simulink model "adm_pcie_9h7_dts_dual_2x100g_dsp"  (R2019a)
settings: Solver=VariableStepAuto  StartTime=0.0  StopTime=10.0  RelTol=1e-3
undefined symbols (not defined in the file): datetime, posixtime
libraries: xbsIndex_r4 x7868, casper_library_misc x12, xps_library x9
(part 4 of 65)

== system adm_pcie_9h7_dts_dual_2x100g_dsp/pipeline0/eq/core5 ==
  note: make up for lack
      | of final FFT reorder
  sync : Inport
  in : Inport  Port=2
  Concat : xbsIndex_r4/Concat  num_inputs=8  dbl_ovrd=off  block_type=concat
  Constant : xbsIndex_r4/Constant  const=1  gui_display_data_type=Boolean  arith_type=Boolean  n_bits=16  bin_pt=14  preci_type=Single  exp_width=8  frac_width=24  explicit_period=on  period=1  equ=P=C  opselect=C  inp2=PCIN>>17  opr=+  inp1=P  carry=CIN  dbl_ovrd=off  block_type=constant
  Constant4 : xbsIndex_r4/Constant  const=0  gui_display_data_type=Fixed-point  arith_type=Unsigned  n_bits=18  bin_pt=0  preci_type=Single  exp_width=8  frac_width=24  explicit_period=on  period=1  equ=P=C  opselect=C  inp2=PCIN>>17  opr=+  inp1=P  carry=CIN  dbl_ovrd=off  block_type=constant
  Constant5 : xbsIndex_r4/Constant  const=0  gui_display_data_type=Fixed-point  arith_type=Boolean  n_bits=1  bin_pt=0  preci_type=Single  exp_width=8  frac_width=24  explicit_period=on  period=1  equ=P=C  opselect=C  inp2=PCIN>>17  opr=+  inp1=P  carry=CIN  dbl_ovrd=off  block_type=constant
  Counter : xbsIndex_r4/Counter  cnt_type=Count Limited  cnt_to=2^nchan * nants - 1  operation=Up  start_count=0  cnt_by_val=1  arith_type=Unsigned  n_bits=ceil(log2(2^nchan * nants))  bin_pt=0  load_pin=off  rst=on  en=off  explicit_period=off  period=1  use_behavioral_HDL=off  implementation=Fabric  use_rpm=on  dbl_ovrd=off  block_type=counter
      settings: xl_area=[0, 0, 0, 0, 0, 0, 0]
  Counter1 : xbsIndex_r4/Counter  cnt_type=Free Running  cnt_to=Inf  operation=Up  start_count=0  cnt_by_val=1  arith_type=Unsigned  n_bits=32  bin_pt=0  load_pin=off  rst=on  en=on  explicit_period=on  period=1  use_behavioral_HDL=off  implementation=Fabric  dbl_ovrd=off  block_type=counter
  Delay2 : xbsIndex_r4/Delay  rst=off  infoeditControl=Selection of Reset will increase slice count due to use of real FFs and instead of SRLs  en=off  latency=1  reg_retiming=on  dbl_ovrd=off  block_type=delay
      settings: xl_area=[0, 0, 0, 0, 0, 0, 0]
  Delay4 : xbsIndex_r4/Delay  rst=off  infoeditControl=Selection of Reset will increase slice count due to use of real FFs and instead of SRLs  en=off  latency=6  reg_retiming=on  dbl_ovrd=off  block_type=delay
      settings: xl_area=[0, 0, 0, 0, 0, 0, 0]
  Delay5 : xbsIndex_r4/Delay  rst=off  infoeditControl=Selection of Reset will increase slice count due to use of real FFs and instead of SRLs  en=off  latency=1  reg_retiming=on  dbl_ovrd=off  block_type=delay
      settings: xl_area=[0, 0, 0, 0, 0, 0, 0]
  Logical : xbsIndex_r4/Logical  logical_function=OR  inputs=8  en=off  latency=1  precision=Full  arith_type=Unsigned  n_bits=16  bin_pt=0  align_bp=on  dbl_ovrd=off  block_type=logical
  bus_expand4 : Subsystem  AncestorBlock=casper_library_flow_control/bus_expand  mask(bus_expand){mode=divisions of equal size, outputNum=8, outputWidth=18*2, outputBinaryPt=0, outputArithmeticType=0, show_format=off, outputToWorkspace=off, variablePrefix=out, outputToModelAsWell=on}
      mask prompts: outputNum "Number of outputs:"; outputWidth "Output width:"; outputBinaryPt "Output binary point position:"; outputArithmeticType "Output arithmetic type (ufix=0, fix=1, bool=2):"; show_format "Print format string?"; outputToWorkspace "Output to workspace?"; variablePrefix "Variable name prefix:"; outputToModelAsWell "Output to model as well?"
      mask help:
      | Expands a 'bus' made using a bus_create or Xilinx
      | concat block.
      | The input will be divided into the specified number
      | of outputs with the specified arithmetic types.
      | Divisions are made from most significant bit.
      mask init: same as adm_pcie_9h7_dts_dual_2x100g_dsp/pipeline0/eq/bus_expand4
      settings: AttributesFormatString=8 outputs
      mask TypeOptions mode: divisions of equal size | divisions of arbitrary size
      mask Callback mode: bus_expand_callback();
      mask Callback outputWidth: bus_expand_callback();
      mask Callback outputToWorkspace: bus_expand_callback();
  clip_cnt : Subsystem  Tag=xps:sw_reg  AncestorBlock=xps_library/Memory/software_register  mask(swreg){io_dir=To Processor, io_delay=0, init_val=0, sample_period=1, names=reg, bitwidths=32, bin_pts=0, arith_types=0, sim_port=on, show_format=on, desc_str=}
      mask prompts: io_dir "I/O direction"; io_delay "I/O delay"; init_val "Initial Value"; sample_period "Sample period"; names "Bitfield names [msb...lsb]"; bitwidths "Bitfield widths"; bin_pts "Bitfield binary pts"; arith_types "Bitfield types, ufix=0, fix=1, bool=2"; sim_port "Provide sim input/output?"; show_format "Print format string?"; desc_str "Description"
      mask help: A 32-bit software-accessible register. Can be divided into bitfields of varying widths and types using the fields in the block mask.
      mask init:
      | swreg_init(gcb)
      settings: AttributesFormatString=1output:uf32.0 = 32 bits
      mask TypeOptions io_dir: To Processor | From Processor
      mask Callback io_dir:
      | mask_enables = get_param(gcb, 'MaskEnables');
      | mask_names = get_param(gcb, 'MaskNames');
      | if strcmp(get_param(gcb, 'io_dir'), 'To Processor'),
      |     mask_enables{ismember(mask_names, 'sample_period')} = 'off';
      | else
      |     mask_enables{ismember(mask_names, 'sample_period')} = 'on';
      | end
      | set_param(gcb, 'MaskEnables', mask_enables);
      mask DialogControl ParameterTabVar0 Prompt: Setup
  coeffs : Subsystem  Tag=xps:bram  AncestorBlock=xps_library/Memory/shared_bram  mask{sample_rate=1, init_vals=[0:2^10-1], data_bin_pt=0, optimization=Minimum_Area, reg_core_output=off, reg_prim_output=off, data_width=16, addr_width=ceil(log2(2^nchan * nants)), arith_type=Unsigned, desc_str=|, type_desc=uint16}
      mask desc_str=|
      | For register name suffix ``<n>_coeffs``, this
      | memory holds coefficients for F-engine streams
      | ``16n..16(n+1)-1``. Coefficients are stored
      | as a ``[16, n_fft_channels / 8]`` array, where the first
      | axis (over input number) varies *slowest*.
      | Coefficients are shared over 8 consecutive frequency
      | channels, with coefficient ``m`` being applied to
      | frequency channel ``m..8(m+1)-1``. Coefficients
      | are interpretted with 5 bits below the binary point.
      mask prompts: sample_rate "Sample rate"; init_vals "Initial values (simulation only)"; data_bin_pt "Data Binary Point"; reg_core_output "Register Core Output"; reg_prim_output "Register Primitive Output"; data_width "Data Width"; addr_width "Address width"; arith_type "Output Data Type"; desc_str "Description"; type_desc "Word Type Description"
      mask init:
      | shared_bram_mask;
      mask TypeOptions optimization: Minimum_Area | Low_Power
      mask TypeOptions data_width: 8 | 16 | 32 | 64 | 128
      mask TypeOptions arith_type: Unsigned | Signed  (2's comp)
      mask DialogControl Container4 Prompt: Configuration
      mask DialogControl Container10 Prompt: Documentation
  round1 : Subsystem
      settings: AttributesFormatString=latency=5
  round2 : Subsystem
      settings: AttributesFormatString=latency=5
  round3 : Subsystem
      settings: AttributesFormatString=latency=5
  round4 : Subsystem
      settings: AttributesFormatString=latency=5
  round5 : Subsystem
      settings: AttributesFormatString=latency=5
  round6 : Subsystem
      settings: AttributesFormatString=latency=5
  round7 : Subsystem
      settings: AttributesFormatString=latency=5
  round8 : Subsystem
      settings: AttributesFormatString=latency=5
  sync_out : Outport
  dout : Outport  Port=2
  wires:
  Delay5/1 -> Delay4/1
  Delay2/1 -> bus_expand4/1(bus_in)
  coeffs/1(data_out) -> round8/2(scale), round7/2(scale), round6/2(scale), round5/2(scale), round4/2(scale), round3/2(scale), round2/2(scale), round1/2(scale)
  in/1 -> Delay2/1
  sync/1 -> Delay5/1, Counter/1
  Constant5/1 -> coeffs/3(we)
  Constant4/1 -> coeffs/2(data_in)
  bus_expand4/3(out6) -> round3/1(din)
  bus_expand4/2(out7) -> round2/1(din)
  bus_expand4/1(msb_out8) -> round1/1(din)
  bus_expand4/4(out5) -> round4/1(din)
  bus_expand4/5(out4) -> round5/1(din)
  bus_expand4/6(out3) -> round6/1(din)
  bus_expand4/7(out2) -> round7/1(din)
  bus_expand4/8(lsb_out1) -> round8/1(din)
  round1/1(dout) -> Concat/1
  round2/1(dout) -> Concat/2
  round3/1(dout) -> Concat/3
  round4/1(dout) -> Concat/4
  round5/1(dout) -> Concat/5
  round6/1(dout) -> Concat/6
  round7/1(dout) -> Concat/7
  round8/1(dout) -> Concat/8
  round1/2(clip) -> Logical/1
  round3/2(clip) -> Logical/3
  round2/2(clip) -> Logical/2
  round6/2(clip) -> Logical/6
  round5/2(clip) -> Logical/5
  round7/2(clip) -> Logical/7
  Logical/1 -> Counter1/2
  round4/2(clip) -> Logical/4
  Counter1/1 -> clip_cnt/1(out_reg)
  round8/2(clip) -> Logical/8
  Concat/1 -> dout/1
  Delay4/1 -> sync_out/1, Counter1/1
  Constant/1 -> ?
  Counter/1 -> coeffs/1(addr)

== system adm_pcie_9h7_dts_dual_2x100g_dsp/pipeline0/eq/core6 ==
  note: make up for lack
      | of final FFT reorder
  sync : Inport
  in : Inport  Port=2
  Concat : xbsIndex_r4/Concat  num_inputs=8  dbl_ovrd=off  block_type=concat
  Constant : xbsIndex_r4/Constant  const=1  gui_display_data_type=Boolean  arith_type=Boolean  n_bits=16  bin_pt=14  preci_type=Single  exp_width=8  frac_width=24  explicit_period=on  period=1  equ=P=C  opselect=C  inp2=PCIN>>17  opr=+  inp1=P  carry=CIN  dbl_ovrd=off  block_type=constant
  Constant4 : xbsIndex_r4/Constant  const=0  gui_display_data_type=Fixed-point  arith_type=Unsigned  n_bits=18  bin_pt=0  preci_type=Single  exp_width=8  frac_width=24  explicit_period=on  period=1  equ=P=C  opselect=C  inp2=PCIN>>17  opr=+  inp1=P  carry=CIN  dbl_ovrd=off  block_type=constant
  Constant5 : xbsIndex_r4/Constant  const=0  gui_display_data_type=Fixed-point  arith_type=Boolean  n_bits=1  bin_pt=0  preci_type=Single  exp_width=8  frac_width=24  explicit_period=on  period=1  equ=P=C  opselect=C  inp2=PCIN>>17  opr=+  inp1=P  carry=CIN  dbl_ovrd=off  block_type=constant
  Counter : xbsIndex_r4/Counter  cnt_type=Count Limited  cnt_to=2^nchan * nants - 1  operation=Up  start_count=0  cnt_by_val=1  arith_type=Unsigned  n_bits=ceil(log2(2^nchan * nants))  bin_pt=0  load_pin=off  rst=on  en=off  explicit_period=off  period=1  use_behavioral_HDL=off  implementation=Fabric  use_rpm=on  dbl_ovrd=off  block_type=counter
      settings: xl_area=[0, 0, 0, 0, 0, 0, 0]
  Counter1 : xbsIndex_r4/Counter  cnt_type=Free Running  cnt_to=Inf  operation=Up  start_count=0  cnt_by_val=1  arith_type=Unsigned  n_bits=32  bin_pt=0  load_pin=off  rst=on  en=on  explicit_period=on  period=1  use_behavioral_HDL=off  implementation=Fabric  dbl_ovrd=off  block_type=counter
  Delay2 : xbsIndex_r4/Delay  rst=off  infoeditControl=Selection of Reset will increase slice count due to use of real FFs and instead of SRLs  en=off  latency=1  reg_retiming=on  dbl_ovrd=off  block_type=delay
      settings: xl_area=[0, 0, 0, 0, 0, 0, 0]
  Delay4 : xbsIndex_r4/Delay  rst=off  infoeditControl=Selection of Reset will increase slice count due to use of real FFs and instead of SRLs  en=off  latency=6  reg_retiming=on  dbl_ovrd=off  block_type=delay
      settings: xl_area=[0, 0, 0, 0, 0, 0, 0]
  Delay5 : xbsIndex_r4/Delay  rst=off  infoeditControl=Selection of Reset will increase slice count due to use of real FFs and instead of SRLs  en=off  latency=1  reg_retiming=on  dbl_ovrd=off  block_type=delay
      settings: xl_area=[0, 0, 0, 0, 0, 0, 0]
  Logical : xbsIndex_r4/Logical  logical_function=OR  inputs=8  en=off  latency=1  precision=Full  arith_type=Unsigned  n_bits=16  bin_pt=0  align_bp=on  dbl_ovrd=off  block_type=logical
  bus_expand4 : Subsystem  AncestorBlock=casper_library_flow_control/bus_expand  mask(bus_expand){mode=divisions of equal size, outputNum=8, outputWidth=18*2, outputBinaryPt=0, outputArithmeticType=0, show_format=off, outputToWorkspace=off, variablePrefix=out, outputToModelAsWell=on}
      mask prompts: outputNum "Number of outputs:"; outputWidth "Output width:"; outputBinaryPt "Output binary point position:"; outputArithmeticType "Output arithmetic type (ufix=0, fix=1, bool=2):"; show_format "Print format string?"; outputToWorkspace "Output to workspace?"; variablePrefix "Variable name prefix:"; outputToModelAsWell "Output to model as well?"
      mask help:
      | Expands a 'bus' made using a bus_create or Xilinx
      | concat block.
      | The input will be divided into the specified number
      | of outputs with the specified arithmetic types.
      | Divisions are made from most significant bit.
      mask init: same as adm_pcie_9h7_dts_dual_2x100g_dsp/pipeline0/eq/bus_expand4
      settings: AttributesFormatString=8 outputs
      mask TypeOptions mode: divisions of equal size | divisions of arbitrary size
      mask Callback mode: bus_expand_callback();
      mask Callback outputWidth: bus_expand_callback();
      mask Callback outputToWorkspace: bus_expand_callback();
  clip_cnt : Subsystem  Tag=xps:sw_reg  AncestorBlock=xps_library/Memory/software_register  mask(swreg){io_dir=To Processor, io_delay=0, init_val=0, sample_period=1, names=reg, bitwidths=32, bin_pts=0, arith_types=0, sim_port=on, show_format=on, desc_str=}
      mask prompts: io_dir "I/O direction"; io_delay "I/O delay"; init_val "Initial Value"; sample_period "Sample period"; names "Bitfield names [msb...lsb]"; bitwidths "Bitfield widths"; bin_pts "Bitfield binary pts"; arith_types "Bitfield types, ufix=0, fix=1, bool=2"; sim_port "Provide sim input/output?"; show_format "Print format string?"; desc_str "Description"
      mask help: A 32-bit software-accessible register. Can be divided into bitfields of varying widths and types using the fields in the block mask.
      mask init:
      | swreg_init(gcb)
      settings: AttributesFormatString=1output:uf32.0 = 32 bits
      mask TypeOptions io_dir: To Processor | From Processor
      mask Callback io_dir:
      | mask_enables = get_param(gcb, 'MaskEnables');
      | mask_names = get_param(gcb, 'MaskNames');
      | if strcmp(get_param(gcb, 'io_dir'), 'To Processor'),
      |     mask_enables{ismember(mask_names, 'sample_period')} = 'off';
      | else
      |     mask_enables{ismember(mask_names, 'sample_period')} = 'on';
      | end
      | set_param(gcb, 'MaskEnables', mask_enables);
      mask DialogControl ParameterTabVar0 Prompt: Setup
  coeffs : Subsystem  Tag=xps:bram  AncestorBlock=xps_library/Memory/shared_bram  mask{sample_rate=1, init_vals=[0:2^10-1], data_bin_pt=0, optimization=Minimum_Area, reg_core_output=off, reg_prim_output=off, data_width=16, addr_width=ceil(log2(2^nchan * nants)), arith_type=Unsigned, desc_str=|, type_desc=uint16}
      mask desc_str=|
      | For register name suffix ``<n>_coeffs``, this
      | memory holds coefficients for F-engine streams
      | ``16n..16(n+1)-1``. Coefficients are stored
      | as a ``[16, n_fft_channels / 8]`` array, where the first
      | axis (over input number) varies *slowest*.
      | Coefficients are shared over 8 consecutive frequency
      | channels, with coefficient ``m`` being applied to
      | frequency channel ``m..8(m+1)-1``. Coefficients
      | are interpretted with 5 bits below the binary point.
      mask prompts: sample_rate "Sample rate"; init_vals "Initial values (simulation only)"; data_bin_pt "Data Binary Point"; reg_core_output "Register Core Output"; reg_prim_output "Register Primitive Output"; data_width "Data Width"; addr_width "Address width"; arith_type "Output Data Type"; desc_str "Description"; type_desc "Word Type Description"
      mask init:
      | shared_bram_mask;
      mask TypeOptions optimization: Minimum_Area | Low_Power
      mask TypeOptions data_width: 8 | 16 | 32 | 64 | 128
      mask TypeOptions arith_type: Unsigned | Signed  (2's comp)
      mask DialogControl Container4 Prompt: Configuration
      mask DialogControl Container10 Prompt: Documentation
  round1 : Subsystem
      settings: AttributesFormatString=latency=5
  round2 : Subsystem
      settings: AttributesFormatString=latency=5
  round3 : Subsystem
      settings: AttributesFormatString=latency=5
  round4 : Subsystem
      settings: AttributesFormatString=latency=5
  round5 : Subsystem
      settings: AttributesFormatString=latency=5
  round6 : Subsystem
      settings: AttributesFormatString=latency=5
  round7 : Subsystem
      settings: AttributesFormatString=latency=5
  round8 : Subsystem
      settings: AttributesFormatString=latency=5
  sync_out : Outport
  dout : Outport  Port=2
  wires:
  Delay5/1 -> Delay4/1
  Delay2/1 -> bus_expand4/1(bus_in)
  coeffs/1(data_out) -> round8/2(scale), round7/2(scale), round6/2(scale), round5/2(scale), round4/2(scale), round3/2(scale), round2/2(scale), round1/2(scale)
  in/1 -> Delay2/1
  sync/1 -> Delay5/1, Counter/1
  Constant5/1 -> coeffs/3(we)
  Constant4/1 -> coeffs/2(data_in)
  bus_expand4/3(out6) -> round3/1(din)
  bus_expand4/2(out7) -> round2/1(din)
  bus_expand4/1(msb_out8) -> round1/1(din)
  bus_expand4/4(out5) -> round4/1(din)
  bus_expand4/5(out4) -> round5/1(din)
  bus_expand4/6(out3) -> round6/1(din)
  bus_expand4/7(out2) -> round7/1(din)
  bus_expand4/8(lsb_out1) -> round8/1(din)
  round1/1(dout) -> Concat/1
  round2/1(dout) -> Concat/2
  round3/1(dout) -> Concat/3
  round4/1(dout) -> Concat/4
  round5/1(dout) -> Concat/5
  round6/1(dout) -> Concat/6
  round7/1(dout) -> Concat/7
  round8/1(dout) -> Concat/8
  round1/2(clip) -> Logical/1
  round3/2(clip) -> Logical/3
  round2/2(clip) -> Logical/2
  round6/2(clip) -> Logical/6
  round5/2(clip) -> Logical/5
  round7/2(clip) -> Logical/7
  Logical/1 -> Counter1/2
  round4/2(clip) -> Logical/4
  Counter1/1 -> clip_cnt/1(out_reg)
  round8/2(clip) -> Logical/8
  Concat/1 -> dout/1
  Delay4/1 -> sync_out/1, Counter1/1
  Constant/1 -> ?
  Counter/1 -> coeffs/1(addr)

== system adm_pcie_9h7_dts_dual_2x100g_dsp/pipeline0/eq/core7 ==
  note: make up for lack
      | of final FFT reorder
  sync : Inport
  in : Inport  Port=2
  Concat : xbsIndex_r4/Concat  num_inputs=8  dbl_ovrd=off  block_type=concat
  Constant : xbsIndex_r4/Constant  const=1  gui_display_data_type=Boolean  arith_type=Boolean  n_bits=16  bin_pt=14  preci_type=Single  exp_width=8  frac_width=24  explicit_period=on  period=1  equ=P=C  opselect=C  inp2=PCIN>>17  opr=+  inp1=P  carry=CIN  dbl_ovrd=off  block_type=constant
  Constant4 : xbsIndex_r4/Constant  const=0  gui_display_data_type=Fixed-point  arith_type=Unsigned  n_bits=18  bin_pt=0  preci_type=Single  exp_width=8  frac_width=24  explicit_period=on  period=1  equ=P=C  opselect=C  inp2=PCIN>>17  opr=+  inp1=P  carry=CIN  dbl_ovrd=off  block_type=constant
  Constant5 : xbsIndex_r4/Constant  const=0  gui_display_data_type=Fixed-point  arith_type=Boolean  n_bits=1  bin_pt=0  preci_type=Single  exp_width=8  frac_width=24  explicit_period=on  period=1  equ=P=C  opselect=C  inp2=PCIN>>17  opr=+  inp1=P  carry=CIN  dbl_ovrd=off  block_type=constant
  Counter : xbsIndex_r4/Counter  cnt_type=Count Limited  cnt_to=2^nchan * nants - 1  operation=Up  start_count=0  cnt_by_val=1  arith_type=Unsigned  n_bits=ceil(log2(2^nchan * nants))  bin_pt=0  load_pin=off  rst=on  en=off  explicit_period=off  period=1  use_behavioral_HDL=off  implementation=Fabric  use_rpm=on  dbl_ovrd=off  block_type=counter
      settings: xl_area=[0, 0, 0, 0, 0, 0, 0]
  Counter1 : xbsIndex_r4/Counter  cnt_type=Free Running  cnt_to=Inf  operation=Up  start_count=0  cnt_by_val=1  arith_type=Unsigned  n_bits=32  bin_pt=0  load_pin=off  rst=on  en=on  explicit_period=on  period=1  use_behavioral_HDL=off  implementation=Fabric  dbl_ovrd=off  block_type=counter
  Delay2 : xbsIndex_r4/Delay  rst=off  infoeditControl=Selection of Reset will increase slice count due to use of real FFs and instead of SRLs  en=off  latency=1  reg_retiming=on  dbl_ovrd=off  block_type=delay
      settings: xl_area=[0, 0, 0, 0, 0, 0, 0]
  Delay4 : xbsIndex_r4/Delay  rst=off  infoeditControl=Selection of Reset will increase slice count due to use of real FFs and instead of SRLs  en=off  latency=6  reg_retiming=on  dbl_ovrd=off  block_type=delay
      settings: xl_area=[0, 0, 0, 0, 0, 0, 0]
  Delay5 : xbsIndex_r4/Delay  rst=off  infoeditControl=Selection of Reset will increase slice count due to use of real FFs and instead of SRLs  en=off  latency=1  reg_retiming=on  dbl_ovrd=off  block_type=delay
      settings: xl_area=[0, 0, 0, 0, 0, 0, 0]
  Logical : xbsIndex_r4/Logical  logical_function=OR  inputs=8  en=off  latency=1  precision=Full  arith_type=Unsigned  n_bits=16  bin_pt=0  align_bp=on  dbl_ovrd=off  block_type=logical
  bus_expand4 : Subsystem  AncestorBlock=casper_library_flow_control/bus_expand  mask(bus_expand){mode=divisions of equal size, outputNum=8, outputWidth=18*2, outputBinaryPt=0, outputArithmeticType=0, show_format=off, outputToWorkspace=off, variablePrefix=out, outputToModelAsWell=on}
      mask prompts: outputNum "Number of outputs:"; outputWidth "Output width:"; outputBinaryPt "Output binary point position:"; outputArithmeticType "Output arithmetic type (ufix=0, fix=1, bool=2):"; show_format "Print format string?"; outputToWorkspace "Output to workspace?"; variablePrefix "Variable name prefix:"; outputToModelAsWell "Output to model as well?"
      mask help:
      | Expands a 'bus' made using a bus_create or Xilinx
      | concat block.
      | The input will be divided into the specified number
      | of outputs with the specified arithmetic types.
      | Divisions are made from most significant bit.
      mask init: same as adm_pcie_9h7_dts_dual_2x100g_dsp/pipeline0/eq/bus_expand4
      settings: AttributesFormatString=8 outputs
      mask TypeOptions mode: divisions of equal size | divisions of arbitrary size
      mask Callback mode: bus_expand_callback();
      mask Callback outputWidth: bus_expand_callback();
      mask Callback outputToWorkspace: bus_expand_callback();
  clip_cnt : Subsystem  Tag=xps:sw_reg  AncestorBlock=xps_library/Memory/software_register  mask(swreg){io_dir=To Processor, io_delay=0, init_val=0, sample_period=1, names=reg, bitwidths=32, bin_pts=0, arith_types=0, sim_port=on, show_format=on, desc_str=}
      mask prompts: io_dir "I/O direction"; io_delay "I/O delay"; init_val "Initial Value"; sample_period "Sample period"; names "Bitfield names [msb...lsb]"; bitwidths "Bitfield widths"; bin_pts "Bitfield binary pts"; arith_types "Bitfield types, ufix=0, fix=1, bool=2"; sim_port "Provide sim input/output?"; show_format "Print format string?"; desc_str "Description"
      mask help: A 32-bit software-accessible register. Can be divided into bitfields of varying widths and types using the fields in the block mask.
      mask init:
      | swreg_init(gcb)
      settings: AttributesFormatString=1output:uf32.0 = 32 bits
      mask TypeOptions io_dir: To Processor | From Processor
      mask Callback io_dir:
      | mask_enables = get_param(gcb, 'MaskEnables');
      | mask_names = get_param(gcb, 'MaskNames');
      | if strcmp(get_param(gcb, 'io_dir'), 'To Processor'),
      |     mask_enables{ismember(mask_names, 'sample_period')} = 'off';
      | else
      |     mask_enables{ismember(mask_names, 'sample_period')} = 'on';
      | end
      | set_param(gcb, 'MaskEnables', mask_enables);
      mask DialogControl ParameterTabVar0 Prompt: Setup
  coeffs : Subsystem  Tag=xps:bram  AncestorBlock=xps_library/Memory/shared_bram  mask{sample_rate=1, init_vals=[0:2^10-1], data_bin_pt=0, optimization=Minimum_Area, reg_core_output=off, reg_prim_output=off, data_width=16, addr_width=ceil(log2(2^nchan * nants)), arith_type=Unsigned, desc_str=|, type_desc=uint16}
      mask desc_str=|
      | For register name suffix ``<n>_coeffs``, this
      | memory holds coefficients for F-engine streams
      | ``16n..16(n+1)-1``. Coefficients are stored
      | as a ``[16, n_fft_channels / 8]`` array, where the first
      | axis (over input number) varies *slowest*.
      | Coefficients are shared over 8 consecutive frequency
      | channels, with coefficient ``m`` being applied to
      | frequency channel ``m..8(m+1)-1``. Coefficients
      | are interpretted with 5 bits below the binary point.
      mask prompts: sample_rate "Sample rate"; init_vals "Initial values (simulation only)"; data_bin_pt "Data Binary Point"; reg_core_output "Register Core Output"; reg_prim_output "Register Primitive Output"; data_width "Data Width"; addr_width "Address width"; arith_type "Output Data Type"; desc_str "Description"; type_desc "Word Type Description"
      mask init:
      | shared_bram_mask;
      mask TypeOptions optimization: Minimum_Area | Low_Power
      mask TypeOptions data_width: 8 | 16 | 32 | 64 | 128
      mask TypeOptions arith_type: Unsigned | Signed  (2's comp)
      mask DialogControl Container4 Prompt: Configuration
      mask DialogControl Container10 Prompt: Documentation
  round1 : Subsystem
      settings: AttributesFormatString=latency=5
  round2 : Subsystem
      settings: AttributesFormatString=latency=5
  round3 : Subsystem
      settings: AttributesFormatString=latency=5
  round4 : Subsystem
      settings: AttributesFormatString=latency=5
  round5 : Subsystem
      settings: AttributesFormatString=latency=5
  round6 : Subsystem
      settings: AttributesFormatString=latency=5
  round7 : Subsystem
      settings: AttributesFormatString=latency=5
  round8 : Subsystem
      settings: AttributesFormatString=latency=5
  sync_out : Outport
  dout : Outport  Port=2
  wires:
  Counter/1 -> coeffs/1(addr)
  Constant/1 -> ?
  Delay4/1 -> Counter1/1, sync_out/1
  Concat/1 -> dout/1
  round8/2(clip) -> Logical/8
  Counter1/1 -> clip_cnt/1(out_reg)
  round4/2(clip) -> Logical/4
  Logical/1 -> Counter1/2
  round7/2(clip) -> Logical/7
  round5/2(clip) -> Logical/5
  round6/2(clip) -> Logical/6
  round2/2(clip) -> Logical/2
  round3/2(clip) -> Logical/3
  round1/2(clip) -> Logical/1
  round8/1(dout) -> Concat/8
  round7/1(dout) -> Concat/7
  round6/1(dout) -> Concat/6
  round5/1(dout) -> Concat/5
  round4/1(dout) -> Concat/4
  round3/1(dout) -> Concat/3
  round2/1(dout) -> Concat/2
  round1/1(dout) -> Concat/1
  bus_expand4/8(lsb_out1) -> round8/1(din)
  bus_expand4/7(out2) -> round7/1(din)
  bus_expand4/6(out3) -> round6/1(din)
  bus_expand4/5(out4) -> round5/1(din)
  bus_expand4/4(out5) -> round4/1(din)
  bus_expand4/1(msb_out8) -> round1/1(din)
  bus_expand4/2(out7) -> round2/1(din)
  bus_expand4/3(out6) -> round3/1(din)
  Constant4/1 -> coeffs/2(data_in)
  Constant5/1 -> coeffs/3(we)
  sync/1 -> Counter/1, Delay5/1
  in/1 -> Delay2/1
  coeffs/1(data_out) -> round1/2(scale), round2/2(scale), round3/2(scale), round4/2(scale), round5/2(scale), round6/2(scale), round7/2(scale), round8/2(scale)
  Delay2/1 -> bus_expand4/1(bus_in)
  Delay5/1 -> Delay4/1
